simulink model "senderBlock"  (R2021b)
settings: Solver=VariableStepAuto  StartTime=0.0  StopTime=10.0  RelTol=1e-3
settings Model: Creator=vgaggero  LastModifiedBy=vgaggero

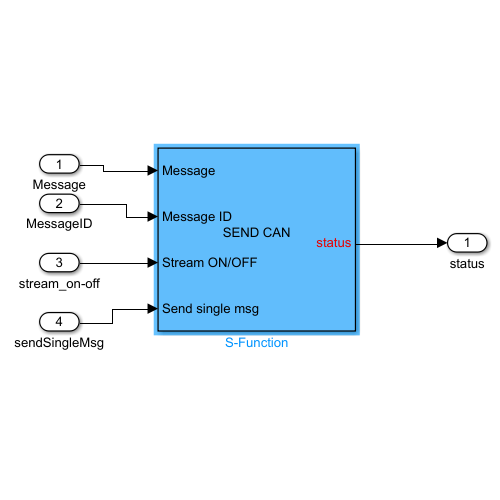
[thumbnail: Simulink's stored preview of the top-level diagram]
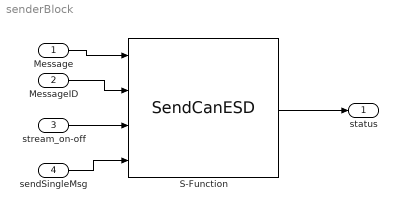
== system senderBlock ==
  Message : Inport  PortDimensions=8
  MessageID : Inport  Port=2  PortDimensions=1
  stream_on-off : Inport  Port=3  PortDimensions=1
  sendSingleMsg : Inport  Port=4  PortDimensions=1
  S-Function : S-Function  FunctionName=SendCanESD  Parameters=(baudrate-1),netid,length, txQueueSize, rxQueueSize, txTimeout, rxTimeout  SFunctionDeploymentMode=off  EnableBusSupport=off  mask{baudrate=1000 Kbit/s, netid=0, length=8, txQueueSize=1, rxQueueSize=1, txTimeout=0, rxTimeout=0}
      mask prompts: netid "CAN Network"; length "Message Length"; txQueueSize "Tx queue size"; rxQueueSize "Rx queue size"; txTimeout "Tx timeout"; rxTimeout "Rx timeout"
      mask TypeOptions baudrate: 1000 Kbit/s | 500 Kbit/s
      mask Display:
      | fprintf('SEND CAN\n')
      | port_label('input',1,'Message');
      | port_label('input',2,'Message ID');
      | port_label('input',3,'Stream ON/OFF');
      | port_label('input',4,'Send single msg');
      | color('red');port_label('output',1,'status');
  status : Outport  PortDimensions=1
  wires:
  S-Function/1 -> status/1
  Message/1 -> S-Function/1
  MessageID/1 -> S-Function/2
  stream_on-off/1 -> S-Function/3
  sendSingleMsg/1 -> S-Function/4
